simulink model "Quadrotor"  (R2018a)
settings: Solver=ode4  StartTime=0.0  StopTime=50  FixedStep=0.001  RelTol=1e-3
libraries: simulink x12
settings Model: Creator=info  LastModifiedBy=oussa

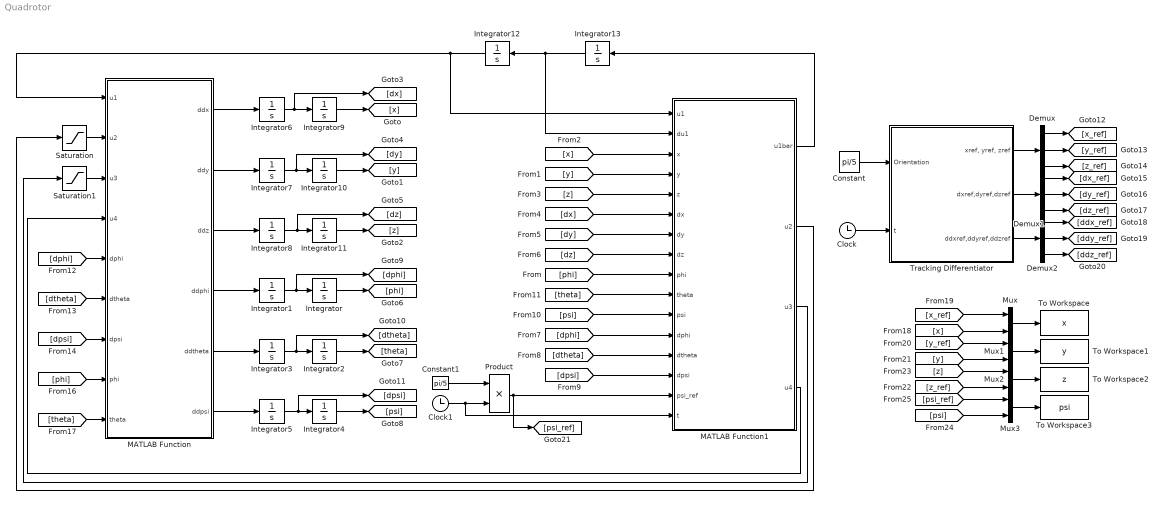
== system Quadrotor ==
  Clock : Clock
  Clock1 : Clock
  Constant : Constant  Value=pi/5
  Constant1 : Constant  Value=pi/5
  Demux : Demux  Outputs=3
  Demux1 : Demux  Outputs=3
  Demux2 : Demux  Outputs=3
  Integrator{,1..13} (14 alike) : Integrator
  MATLAB Function : MATLAB Function  TreatAsAtomicUnit=on
  MATLAB Function1 : MATLAB Function  TreatAsAtomicUnit=on
  Mux{,1..3} (4 alike) : Mux  Inputs=2
  Product : Product
  Saturation : Saturate  UpperLimit=inf  LowerLimit=-inf
  Saturation1 : Saturate  UpperLimit=inf  LowerLimit=-inf
  To Workspace : ToWorkspace  VariableName=x  SaveFormat=Timeseries  SampleTime=-1
  To Workspace1 : ToWorkspace  VariableName=y  SaveFormat=Timeseries  SampleTime=-1
  To Workspace2 : ToWorkspace  VariableName=z  SaveFormat=Timeseries  SampleTime=-1
  To Workspace3 : ToWorkspace  VariableName=psi  SaveFormat=Timeseries  SampleTime=-1
  Tracking Differentiator : Subsystem
  wires:
  MATLAB Function/4(ddphi) -> Integrator1/1
  Integrator1/1 -> [dphi], Integrator/1
  Integrator3/1 -> [dtheta], Integrator2/1
  MATLAB Function/5(ddtheta) -> Integrator3/1
  MATLAB Function/6(ddpsi) -> Integrator5/1
  MATLAB Function/1(ddx) -> Integrator6/1
  MATLAB Function/2(ddy) -> Integrator7/1
  MATLAB Function/3(ddz) -> Integrator8/1
  Integrator6/1 -> [dx], Integrator9/1
  Integrator7/1 -> [dy], Integrator10/1
  Integrator8/1 -> [dz], Integrator11/1
  Integrator13/1 -> Integrator12/1, MATLAB Function1/2(du1)
  Integrator12/1 -> MATLAB Function/1(u1), MATLAB Function1/1(u1)
  Integrator9/1 -> [x]
  Integrator10/1 -> [y]
  [y] -> MATLAB Function1/4(y)
  [z] -> MATLAB Function1/5(z)
  Integrator11/1 -> [z]
  Integrator/1 -> [phi]
  Integrator4/1 -> [psi]
  Integrator2/1 -> [theta]
  [phi] -> MATLAB Function1/9(phi)
  Integrator5/1 -> [dpsi], Integrator4/1
  [dy] -> MATLAB Function1/7(dy)
  [dz] -> MATLAB Function1/8(dz)
  [dtheta] -> MATLAB Function1/13(dtheta)
  [dpsi] -> MATLAB Function1/14(dpsi)
  [theta] -> MATLAB Function1/10(theta)
  MATLAB Function1/2(u2) -> Saturation/1
  MATLAB Function1/3(u3) -> Saturation1/1
  MATLAB Function1/4(u4) -> MATLAB Function/4(u4)
  [dphi] -> MATLAB Function/5(dphi)
  [dtheta] -> MATLAB Function/6(dtheta)
  [dpsi] -> MATLAB Function/7(dpsi)
  [phi] -> MATLAB Function/8(phi)
  [theta] -> MATLAB Function/9(theta)
  Constant/1 -> Tracking Differentiator/1(Orientation)
  Clock/1 -> Tracking Differentiator/2(t)
  Product/1 -> MATLAB Function1/15(psi_ref), [psi_ref]
  Constant1/1 -> Product/1
  Clock1/1 -> MATLAB Function1/16(t), Product/2
  Tracking Differentiator/1("xref, yref, zref") -> Demux/1
  Demux/1 -> [x_ref]
  Demux/2 -> [y_ref]
  Demux/3 -> [z_ref]
  Demux1/3 -> [dz_ref]
  Demux1/2 -> [dy_ref]
  Demux1/1 -> [dx_ref]
  Tracking Differentiator/2(dxref,dyref,dzref) -> Demux1/1
  Demux2/1 -> [ddx_ref]
  Demux2/2 -> [ddy_ref]
  Demux2/3 -> [ddz_ref]
  Tracking Differentiator/3(ddxref,ddyref,ddzref) -> Demux2/1
  [x] -> Mux/2
  [x_ref] -> Mux/1
  [y_ref] -> Mux1/1
  [y] -> Mux1/2
  [z] -> Mux2/1
  [z_ref] -> Mux2/2
  [psi_ref] -> Mux3/1
  [psi] -> Mux3/2
  Saturation/1 -> MATLAB Function/2(u2)
  Saturation1/1 -> MATLAB Function/3(u3)
  MATLAB Function1/1(u1bar) -> Integrator13/1
  [dx] -> MATLAB Function1/6(dx)
  [dphi] -> MATLAB Function1/12(dphi)
  [psi] -> MATLAB Function1/11(psi)
  [x] -> MATLAB Function1/3(x)
  Mux/1 -> To Workspace/1
  Mux1/1 -> To Workspace1/1
  Mux2/1 -> To Workspace2/1
  Mux3/1 -> To Workspace3/1

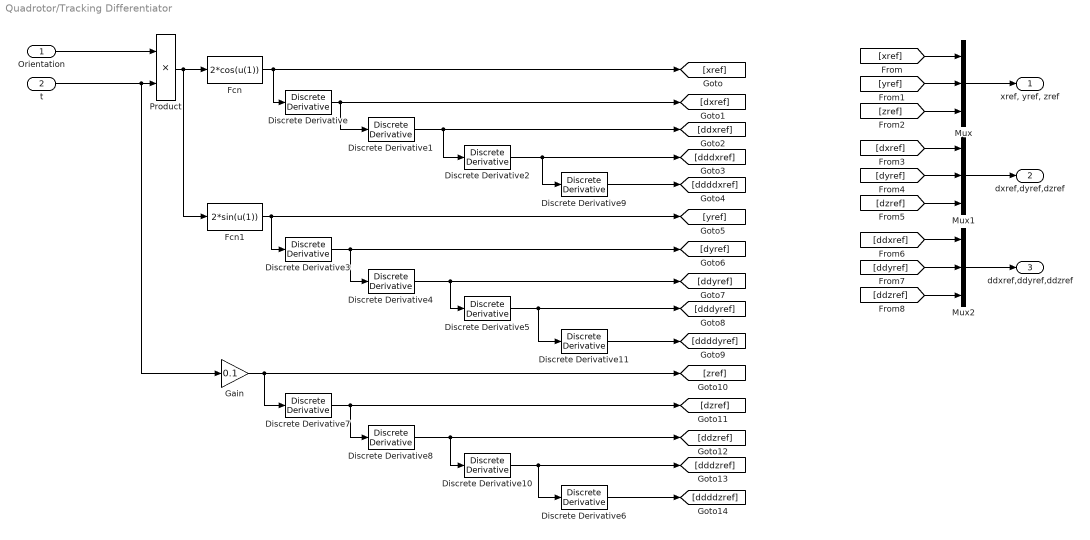
== system Quadrotor/Tracking Differentiator ==
  Orientation : Inport
  t : Inport  Port=2
  Discrete Derivative{,1..11} (12 alike) : simulink/Discrete/Discrete Derivative  gainval=1.0  ICPrevScaledInput=0.0  OutMin=[]  OutMax=[]  OutDataType=fixdt(1, 16)  OutScaling=2^-10  DoSatur=off
  Fcn : Fcn  Expr=2*cos(u(1))
  Fcn1 : Fcn  Expr=2*sin(u(1))
  Gain : Gain  Gain=0.1
  Mux : Mux  Inputs=3
  Mux1 : Mux  Inputs=3
  Mux2 : Mux  Inputs=3
  Product : Product
  "xref, yref, zref" : Outport
  dxref,dyref,dzref : Outport  Port=2
  ddxref,ddyref,ddzref : Outport  Port=3
  wires:
  Product/1 -> Fcn1/1, Fcn/1
  Fcn/1 -> [xref], Discrete Derivative/1
  t/1 -> Gain/1, Product/2
  Orientation/1 -> Product/1
  Discrete Derivative/1 -> [dxref], Discrete Derivative1/1
  Discrete Derivative1/1 -> [ddxref], Discrete Derivative2/1
  Discrete Derivative2/1 -> [dddxref], Discrete Derivative9/1
  Discrete Derivative4/1 -> [ddyref], Discrete Derivative5/1
  Discrete Derivative3/1 -> [dyref], Discrete Derivative4/1
  Discrete Derivative9/1 -> [ddddxref]
  Fcn1/1 -> [yref], Discrete Derivative3/1
  Discrete Derivative5/1 -> [dddyref], Discrete Derivative11/1
  Discrete Derivative11/1 -> [ddddyref]
  Discrete Derivative6/1 -> [ddddzref]
  Discrete Derivative10/1 -> [dddzref], Discrete Derivative6/1
  Gain/1 -> [zref], Discrete Derivative7/1
  Discrete Derivative7/1 -> [dzref], Discrete Derivative8/1
  Discrete Derivative8/1 -> [ddzref], Discrete Derivative10/1
  [xref] -> Mux/1
  [yref] -> Mux/2
  [zref] -> Mux/3
  [dzref] -> Mux1/3
  [dyref] -> Mux1/2
  [dxref] -> Mux1/1
  [ddxref] -> Mux2/1
  [ddyref] -> Mux2/2
  [ddzref] -> Mux2/3
  Mux/1 -> "xref, yref, zref"/1
  Mux1/1 -> dxref,dyref,dzref/1
  Mux2/1 -> ddxref,ddyref,ddzref/1

== matlab function Quadrotor/MATLAB Function1 ==
  data: u1 input; du1 input; x input; y input; z input; dx input; dy input; dz input; u1bar output; phi input; theta input; psi input; dphi input; dtheta input; dpsi input; u2 output; u3 output; u4 output; psi_ref input; t input
function [u1bar,u2,u3,u4] = Feedback_Linearization(u1,du1,x,y,z,dx,dy,dz,phi,theta,psi,dphi,dtheta,dpsi,psi_ref,t)
m = 0.56;g = 9.8; ix = 0.0142; iy = ix; iz = 2*ix;
a1 = (iy-iz)/ix; a2 = (iz-ix)/iy; a3 = (ix-iy)/iz;
b1 = 1/ix; b2 = 1/iy; b3 = 1/iz;
%% High order derivatives of the output
ddx = theta*u1/m;
ddy = -phi*u1/m;
ddz = -g+u1/m;

dddx = dtheta*u1/m+theta*du1/m;
dddy = -dphi*u1/m-phi*du1/m;
dddz = du1/m;
%% Feedback control with poles placement
% A1 = [0 1 0 0;0 0 1 0;0 0 0 1;0 0 0 0]; B1 = [0;0;0;1];
% A2 = A1; B2 = B1;
% A3 = A1; B3 = B1;
% A4 = [0 1;0 0]; B4 = [0;1];
% 
% poles1 = [-2;-2.5;-3;-3.5];
% poles2 = [-2;-2.5;-3;-3.5];
% poles3 = [-2;-2.5;-3;-3.5];
% poles4 = [-2;-2.5];

K1 = [52.5000   79.7500   44.7500   11.0000];
K2 = [52.5000   79.7500   44.7500   11.0000];
K3 = [52.5000   79.7500   44.7500   11.0000];
K4 = [5.0000    4.5000];

%% Reference trajectory

ksi_ref = [2*cos(psi_ref);2*sin(psi_ref);0.1*t];
dksi_ref = [-2*pi/5*sin(psi_ref);2*pi/5*cos(psi_ref);0.1]; dpsi_ref = pi/5;
ddksi_ref = [-2*(pi/5)^2*cos(psi_ref);-2*(pi/5)^2*sin(psi_ref);0]; ddpsi_ref = 0;
dddksi_ref = [2*(pi/5)^3*sin(psi_ref);-2*(pi/5)^3*cos(psi_ref);0];
ddddksi_ref = [2*(pi/5)^4*cos(psi_ref);2*(pi/5)^4*sin(psi_ref);0];


v1 = -K1*[x-ksi_ref(1);dx-dksi_ref(1);ddx-ddksi_ref(1);dddx-dddksi_ref(1)]+ddddksi_ref(1);
v2 = -K2*[y-ksi_ref(2);dy-dksi_ref(2);ddy-ddksi_ref(2);dddy-dddksi_ref(2)]+ddddksi_ref(2);
v3 = -K3*[z-ksi_ref(3);dz-dksi_ref(3);ddz-ddksi_ref(3);dddz-dddksi_ref(3)]+ddddksi_ref(3);
v = [v1;v2;v3];
v4 = -K4*[psi-psi_ref;dpsi-dpsi_ref]+ddpsi_ref;

v = [v;v4];

%% Control law 
% I/O Decoupling and Linearization
delta0 = [2*dtheta*du1/m+a2*u1*dphi*dpsi/m;-2*dphi*du1/m-a1*u1*dtheta*dpsi/m;0;a3*dtheta*dphi];
delta = [theta/m 0 u1*b2/m 0;-phi/m -u1*b1/m 0 0;1/m 0 0 0;0 0 0 b3];


u = pinv(delta)*(-delta0+v);

u1bar = u(1);
u2 = u(2);
u3 = u(3);
u4 = u(4);
end

== matlab function Quadrotor/MATLAB Function ==
  data: ddx output; ddy output; ddz output; ddphi output; ddtheta output; ddpsi output; u1 input; u2 input; u3 input; u4 input; dphi input; dtheta input; dpsi input; phi input; theta input
function [ddx,ddy,ddz,ddphi,ddtheta,ddpsi] = Quadrirotor_model(u1,u2,u3,u4,dphi,dtheta,dpsi,phi,theta)
m = 0.56;g = 9.8; ix = 0.0142; iy = ix; iz = 2*ix;
a1 = (iy-iz)/ix; a2 = (iz-ix)/iy; a3 = (ix-iy)/iz;
b1 = 1/ix; b2 = 1/iy; b3 = 1/iz;

ddx = theta*u1/m;
ddy = -phi*u1/m;
ddz = -g+u1/m;

ddphi = a1*dtheta*dpsi+b1*u2;
ddtheta = a2*dphi*dpsi+b2*u3;
ddpsi = a3*dtheta*dphi+b3*u4;

end
